simulink library "Lib_Thermo_Temp2Enth_TMATS_org"  (Simulink 10.0)
settings: Solver=ode45  StartTime=0.0  StopTime=10.0  RelTol=1e-3  EnableMultiTasking=on
Description:
  | Thomas Modules
settings Model: Creator=jwchapm2  LastModifiedBy=annonymous

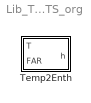
== system Lib_Thermo_Temp2Enth_TMATS_org ==
  Temp2Enth : Subsystem  mask(T-MATS: Temp2Enth Library Block){}
      mask help: This block emperically calculates enthalpy (h) from temperature (T) and fuel to air ratio (FAR).
      mask Help: web(which('Thermo_TMATS_Temp2Enth.html'),'-helpbrowser')

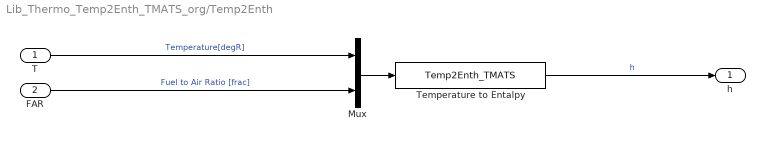
== system Lib_Thermo_Temp2Enth_TMATS_org/Temp2Enth ==
  T : Inport
  FAR : Inport  Port=2
  Mux : Mux  Inputs=2
  Temperature to Entalpy : S-Function  FunctionName=Temp2Enth_TMATS  SFunctionModules='t2hc_TMATS'  SFunctionDeploymentMode=off  EnableBusSupport=off
  h : Outport
  wires:
  Temperature to Entalpy/1 -> h/1  "h"
  Mux/1 -> Temperature to Entalpy/1
  T/1 -> Mux/1  "Temperature[degR]"
  FAR/1 -> Mux/2  "Fuel to Air Ratio [frac]"
